simulink model "w3_warplab_trigger_proc"  (Simulink 7.7)
settings: Solver=ode45  StartTime=0.0  StopTime=100  RelTol=1e-3
InitFcn:
  | warplab_trigger_proc_init
StartFcn:
  | warplab_trigger_proc_init
undefined symbols (not defined in the file or in its folder): gcbh, xlBlockLoadCallback, xlGetNormalizedPeriod
libraries: xbsIndex_r4 x817, xbsEDKLib_r4 x1
(part 1 of 6)
settings Model: Creator=murphpo  LastModifiedBy=chunter
settings DebuggingCC: FcnCallInpInsideContextMsg=Enable All

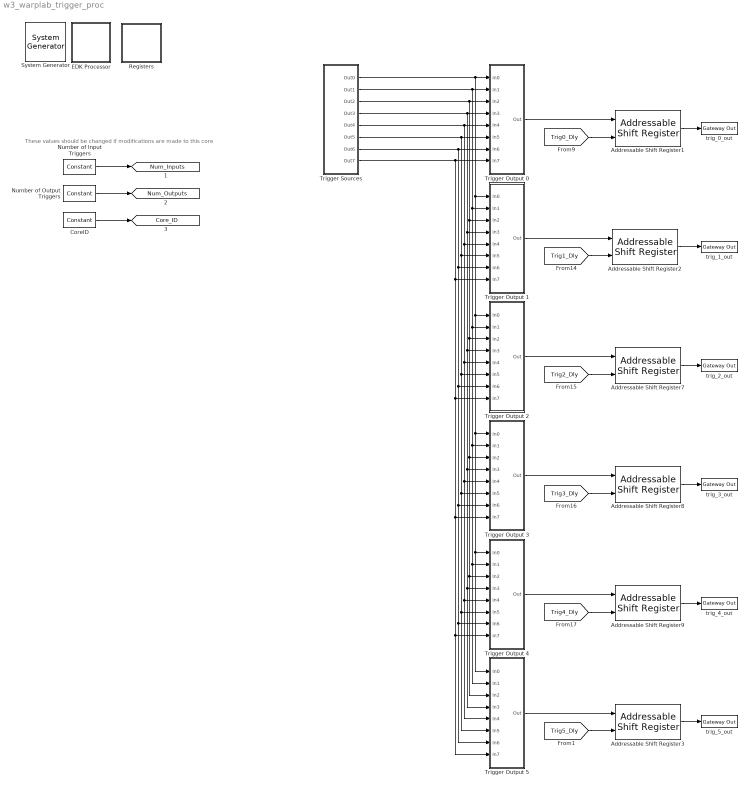
== system w3_warplab_trigger_proc ==
  note: These values should be changed if modifications are made to this core
  " System Generator" : xbsIndex_r4/ System Generator  Tag=genX  SystemSampleTime=-1  xilinxfamily=virtex6  part=xc6vlx240t  speed=-2  package=ff1156  synthesis_tool=XST  clock_wrapper=Clock Enables  directory=./netlist  proj_type=Project Navigator  Synth_file=XST Defaults  Impl_file=ISE Defaults  testbench=off  simulink_period=1  sysclk_period=10  dcm_input_clock_period=10  incr_netlist=off  trim_vbits=Everywhere in SubSystem  dbl_ovrd=According to Block Masks  core_generation=According to Block Masks  run_coregen=off  deprecated_control=off  eval_field=0  block_type=sysgen
  Addressable Shift Register{1..3,7..9} (6 alike) : xbsIndex_r4/Addressable Shift Register  infer_latency=off  depth=32  initVector=[0]  en=off  dbl_ovrd=off  use_behavioral_HDL=off  Optimization=Resource  block_type=addrsr
      settings: infoedit="Delay of configurable length.  Any element in the delay line can be addressed and driven onto the output port.<br><br>Hardware notes: This block is implemented using SRL16s. If Virtex-4 or Spartan-3 device is used, multiple SRLC16s are cascaded together."
  CoreID : xbsIndex_r4/Constant  const=0  gui_display_data_type=Fixed-point  arith_type=Unsigned  n_bits=8  bin_pt=0  preci_type=Single  exp_width=8  frac_width=24  explicit_period=on  period=1  equ=P=C  opselect=C  inp2=PCIN>>17  opr=+  inp1=P  carry=CIN  dbl_ovrd=off  block_type=constant
  EDK Processor : Subsystem  LoadFcn=xlBlockLoadCallback(gcbh);  mask(Xilinx EDK Processor Block){mode=EDK pcore generation, xmp=, MemVisToProc=<qt bgcolor="#FFFFFF"><div><img src="C:/Xilinx/14.4/ISE_DS/ISE/sysgen/data/images/registerplus.gif"> &lt;&lt;RSSI_PKT_DET_CONFIG&gt;&gt;<br></div><div><img src="C:/Xilinx/14.4/ISE_DS/ISE/sysgen/data/images/registerplus.gif"> &lt;&lt;TRIG_CONF_OUT5&gt;&gt;<br></div><div><img src="C:/Xilinx/14.4/ISE_DS/ISE/sysgen/data/images/registerplus.gif"> &lt;&lt;TRIG_CONF_OUT4&gt;&gt;<br></div><div><img src="C:/Xilinx/14.4/ISE_DS/ISE/sysgen/data/images/registerplus.gif"> &lt;&lt;TRIG_CONF_OUT3&gt;&gt;<br></div><div><img src="C:/Xilinx/14.4/ISE_DS/ISE/sysgen/data/images/registerplus.gif"> &lt;&lt;TRIG_CONF_OUT2&gt;&gt;<br></div><div><img src="C:/Xilinx/14.4/ISE_DS/ISE/sysgen/data/images/registerplus.gif"> &lt;&lt;TRIG_CONF_OUT1&gt;&gt;<br></div><div><img src="C:/Xilinx/14.4/ISE_DS/ISE/sysgen/data/images/registerplus.gif"> &lt;&lt;TRIG_CONF_OUT0&gt;&gt;<br></div><div><img src="C:/Xilinx/14.4/ISE_DS/ISE/sysgen/data/images/registerplus.gif"> &lt;&lt;RSSI_PKT_DET_DURATIONS&gt;&gt;<br></div><div><img src="C:/Xilinx/14.4/ISE_DS/ISE/sysgen/data/images/registerplus.gif"> &lt;&lt;RSSI_PKT_DET_THRESHOLDS&gt;&gt;<br></div><div><img src="C:/Xilinx/14.4/ISE_DS/ISE/sysgen/data/images/registerplus.gif"> &lt;&lt;TRIG_CONF_INBANK0&gt;&gt;<br></div><div><img src="C:/Xilinx/14.4/ISE_DS/ISE/sysgen/data/images/registerplus.gif"> &lt;&lt;TRIG_CONF_INBANK1&gt;&gt;<br></div><div><img src="C:/Xilinx/14.4/ISE_DS/ISE/sysgen/data/images/registerplus.gif"> &lt;&lt;CORE_INFO&gt;&gt;<br></div><div><img src="C:/Xilinx/14.4/ISE_DS/ISE/sysgen/data/images/registerplus.gif"> &lt;&lt;TRIG_OUT&gt;&gt;<br></div><div><img src="C:/Xilinx/14.4/ISE_DS/ISE/sysgen/data/images/memoryplus.gif"> &lt;&lt;PktOps0&gt;&gt;<br></div><div><img src="C:/Xilinx/14.4/ISE_DS/ISE/sysgen/data/images/memoryplus.gif"> &lt;&lt;PktTemplate0&gt;&gt;<br></div></qt>, AvailableMemories=<empty>, portInterfaceTable={'exposed'=>[],'portdir'=>[],'portname'=>[],'shortname'=>[]}, bus_type_sgadvanced=, bus_type=AXI, baseaddr=0x80000000, baseaddr_lock_sgadvanced=, baseaddr_lock=off, dual_clock_sgadvanced=, dual_clock=on, reg_readback_sgadvanced=, reg_readback=on, ucf_file=, inheritDeviceType_sgadvanced=, inheritDeviceType=off, elf_file=, codebug_sgadvanced=, codebug=on, clock_name=plb, internalPortList={}, resetPolarity=0, memxtable={'mladdr'=>[0.00000000000000000,1.00000000000000000,2.00000000000000000,3.00000000000000000,4.00000000000000000,5.00000000000000000,6.00000000000000000,7.00000000000000000,8.00000000000000000,9.00000000000000000,10.00000000000000000,0.00000000000000000,1.00000000000000000,-1.00000000000000000,-1.00000000000000000],'mlist'=>['w3_warplab_trigger_proc/Registers/From Register9','w3_warplab_trigger_proc/Registers/From Register7','w3_warplab_trigger_proc/Registers/From Register6','w3_warplab_trigger_proc/Registers/From Register5','w3_warplab_trigger_proc/Registers/From Register4','w3_warplab_trigger_proc/Registers/From Register3','w3_warplab_trigger_proc/Registers/From Register2','w3_warplab_trigger_proc/Registers/From Register11','w3_warplab_trigger_proc/Registers/From Register10','w3_warplab_trigger_proc/Registers/From Register1','w3_warplab_trigger_proc/Registers/From Register','w3_warplab_trigger_proc/Registers/To Register1','w3_warplab_trigger_proc/Registers/To Register','w3_warplab_trigger_proc/Trigger Sources/Ethernet/Pkt Comp/Word Comp 0/Shared Memory2','w3_warplab_trigger_proc/Trigger Sources/Ethernet/Pkt Comp/Word Comp 0/Shared Memory1'],'mlname'=>['\\'RSSI_PKT_DET_CONFIG\\'','\\'TRIG_CONF_OUT5\\'','\\'TRIG_CONF_OUT4\\'','\\'TRIG_CONF_OUT3\\'','\\'TRIG_CONF_OUT2\\'','\\'TRIG_CONF_OUT1\\'','\\'TRIG_CONF_OUT0\\'','\\'RSSI_PKT_DET_DURATIONS\\'','\\'RSSI_PKT_DET_THRESHOLDS\\'','\\'TRIG_CONF_INBANK0\\'','\\'TRIG_CONF_INBANK1\\'','\\'CORE_INFO\\'','\\'TRIG_OUT\\'','\\'PktOps0\\'','\\'PktTemplate0\\''],'mlstate'=>[0.00000000000000000,0.00000000000000000,0.00000000000000000,0.00000000000000000,0.00000000000000000,0.00000000000000000,0.00000000000000000,0.00000000000000000,0.00000000000000000,0.00000000000000000,0.00000000000000000,0.00000000000000000,0.00000000000000000,0.00000000000000000,0.00000000000000000]}, procinfo={}, memmapdirty=off, blockname=, xpsintstyle=default, has_advanced_control=0, sggui_pos=-1,-1,-1,-1, block_type=edkprocessor, block_version=2.7, sg_icon_stat=62,64,-1,-1,white,blue,0,07734,right,,[ ],[ ], sg_mask_display=|, sg_list_contents={'table'=>{'AvailableMemories'=>'popup(<empty>)'}}, sg_blockgui_xml=}
      mask sg_mask_display=|
      | fprintf('','COMMENT: begin icon graphics');
      | patch([0 62 62 0 0 ],[0 0 64 64 0 ],[0.77 0.82 0.91 ]);
      | plot([0 62 62 0 0 ],[0 0 64 64 0 ]);
      | patch([13.2 24.76 32.76 40.76 48.76 32.76 21.2 13.2 ],[40.88 40.88 48.88 40.88 48.88 48.88 48.88 40.88 ],[1 1 1 ]);
      | patch([21.2 32.76 24.76 13.2 21.2 ],[32.88 32.88 40.88 40.88 32.88 ],[0.931 0.946 0.973 ]);
      | patch([13.2 24.76 32.76 21.2 13.2 ],[24.88 24.88 32.88 32.88 24.88 ],[1 1 1 ]);
      | patch([21.2 48.76 40.76 32.76 24.76 13.2 21.2 ],[16.88 16.88 24.88 16.88 24.88 24.88 16.88 ],[0.931 0.946 0.973 ]);
      | fprintf('','COMMENT: end icon graphics');
      | fprintf('','COMMENT: begin icon text');
      | fprintf('','COMMENT: end icon text');
      mask prompts: mode "Configure Processor for"; xmp "XPS Project"; MemVisToProc ""; AvailableMemories "Available Memories"; portInterfaceTable ""; bus_type_sgadvanced ""; bus_type "Bus Type"; baseaddr "Base Address"; baseaddr_lock_sgadvanced ""; baseaddr_lock "Lock"; dual_clock_sgadvanced ""; dual_clock "Dual Clocks"; reg_readback_sgadvanced ""; reg_readback "Register Read-Back"; ucf_file "Constraint File"; inheritDeviceType_sgadvanced ""; inheritDeviceType "Inherit Device Type"; elf_file "Initial Program"; codebug_sgadvanced ""; codebug "Enable Co-Debug with Xilinx SDK (Beta)"; clock_name ""; internalPortList ""; resetPolarity ""; memxtable ""; procinfo ""; memmapdirty ""; blockname ""; xpsintstyle ""; has_advanced_control ""; sggui_pos ""; block_type ""; block_version ""; sg_icon_stat ""; sg_mask_display ""; sg_list_contents ""; sg_blockgui_xml ""
      mask help: Xilinx EDK Processor
      mask init:
      | try
      |   tmp_gcb = gcb;
      |   tmp_gcbh = gcbh;
      |   if (strcmp('SysGenIndex',get_param(bdroot(tmp_gcbh),'tag')) && ~isempty(regexp(bdroot(tmp_gcb), '^xbs', 'once')))
      |     return;
      |   end;
      |   xlMungeMaskParams;
      | 
      |   block_type='edkprocessor';
      | 
      |   serialized_declarations = '{''block_type''=>''String''}';
      |   xledkprocessor_init();
      |   ptable_ = xlblockprep(get_param(tmp_gcb, 'MaskWSVariables'));
      |   try
      |     xlBlockMoveCallback(tmp_gcbh);
      |   catch 
      |      clear global xl_updateicon_recursion_guard;
      |   end;
      | catch
      |   global dbgsysgen;
      |   if(~isempty(dbgsysgen) && dbgsysgen)
      |     e = regexprep(lasterr, '\n', '\nError: ');
      |     disp(['Error: While running MaskInit code on block ' tmp_gcb ': ' e]);
      |     error(e);
      |   end
      | end
      settings: CopyFcn=xlProcBlockCopyCallback(gcbh);xlBlockMoveCallback(gcbh);  DeleteFcn=xlDestroyGui(gcbh);  ModelCloseFcn=xlDestroyGui(gcbh);  PreSaveFcn=xlBlockPreSaveCallback(gcbh);  PostSaveFcn=xlBlockPostSaveCallback(gcbh);  DestroyFcn=xlDestroyGui(gcbh);  OpenFcn=bh=gcbh;xlProcBlockCallbacks('populatesharedmemorylistbox',bh);xlOpenGui(bh, 'edkprocessor_gui.xml', @xlProcBlockEnablement, @xlProcBlockAction);  CloseFcn=xlDestroyGui(gcbh);  MoveFcn=xlBlockMoveCallback(gcbh);
      mask Help: eval('');xlDoc('-book','sysgen','-topic','EDK_Processor');
      mask StyleString: popup(EDK pcore generation|HDL netlisting),edit,edit,edit,edit,edit,popup(AXI|PLB),edit,edit,checkbox,edit,checkbox,edit,checkbox,edit,edit,checkbox,edit,edit,checkbox,edit,edit,edit,edit,edit,edit,edit,edit,edit,edit,edit,edit,edit,edit,edit,edit
      mask Display:
      | fprintf('','COMMENT: begin icon graphics');
      | patch([0 62 62 0 0 ],[0 0 64 64 0 ],[0.77 0.82 0.91 ]);
      | plot([0 62 62 0 0 ],[0 0 64 64 0 ]);
      | patch([13.2 24.76 32.76 40.76 48.76 32.76 21.2 13.2 ],[40.88 40.88 48.88 40.88 48.88 48.88 48.88 40.88 ],[1 1 1 ]);
      | patch([21.2 32.76 24.76 13.2 21.2 ],[32.88 32.88 40.88 40.88 32.88 ],[0.931 0.946 0.973 ]);
      | patch([13.2 24.76 32.76 21.2 13.2 ],[24.88 24.88 32.88 32.88 24.88 ],[1 1 1 ]);
      | patch([21.2 48.76 40.76 32.76 24.76 13.2 21.2 ],[16.88 16.88 24.88 16.88 24.88 24.88 16.88 ],[0.931 0.946 0.973 ]);
      | fprintf('','COMMENT: end icon graphics');
      | fprintf('','COMMENT: begin icon text');
      | disp('');
      | 
      | fprintf('','COMMENT: end icon text');
  Number of Input Triggers : xbsIndex_r4/Constant  const=8  gui_display_data_type=Fixed-point  arith_type=Unsigned  n_bits=8  bin_pt=0  preci_type=Single  exp_width=8  frac_width=24  explicit_period=on  period=1  equ=P=C  opselect=C  inp2=PCIN>>17  opr=+  inp1=P  carry=CIN  dbl_ovrd=off  block_type=constant
  Number of Output Triggers : xbsIndex_r4/Constant  const=6  gui_display_data_type=Fixed-point  arith_type=Unsigned  n_bits=8  bin_pt=0  preci_type=Single  exp_width=8  frac_width=24  explicit_period=on  period=1  equ=P=C  opselect=C  inp2=PCIN>>17  opr=+  inp1=P  carry=CIN  dbl_ovrd=off  block_type=constant
  Registers : Subsystem
  Trigger Output 0 : Subsystem
  Trigger Output 1 : Subsystem
  Trigger Output 2 : Subsystem
  Trigger Output 3 : Subsystem
  Trigger Output 4 : Subsystem
  Trigger Output 5 : Subsystem
  Trigger Sources : Subsystem
  trig_0_out : xbsIndex_r4/Gateway Out  inherit_from_input=off  hdl_port=on  timing_constraint=None  locs_specified=off  LOCs={}  UseAsDAC=off  DACChannel='1'  block_type=gatewayout
  trig_1_out : xbsIndex_r4/Gateway Out  inherit_from_input=off  hdl_port=on  timing_constraint=None  locs_specified=off  LOCs={}  UseAsDAC=off  DACChannel='1'  block_type=gatewayout
  trig_2_out : xbsIndex_r4/Gateway Out  inherit_from_input=off  hdl_port=on  timing_constraint=None  locs_specified=off  LOCs={}  UseAsDAC=off  DACChannel='1'  block_type=gatewayout
  trig_3_out : xbsIndex_r4/Gateway Out  inherit_from_input=off  hdl_port=on  timing_constraint=None  locs_specified=off  LOCs={}  UseAsDAC=off  DACChannel='1'  block_type=gatewayout
  trig_4_out : xbsIndex_r4/Gateway Out  inherit_from_input=off  hdl_port=on  timing_constraint=None  locs_specified=off  LOCs={}  UseAsDAC=off  DACChannel='1'  block_type=gatewayout
  trig_5_out : xbsIndex_r4/Gateway Out  inherit_from_input=off  hdl_port=on  timing_constraint=None  locs_specified=off  LOCs={}  UseAsDAC=off  DACChannel='1'  block_type=gatewayout
  tag scope: Core_ID=global, Num_Inputs=global, Num_Outputs=global
  wires:
  Trigger Sources/1(Out0) -> Trigger Output 0/1(In0), Trigger Output 3/1(In0), Trigger Output 4/1(In0), Trigger Output 5/1(In0), Trigger Output 2/1(In0), Trigger Output 1/1(In0)
  Trigger Sources/2(Out1) -> Trigger Output 0/2(In1), Trigger Output 3/2(In1), Trigger Output 4/2(In1), Trigger Output 5/2(In1), Trigger Output 2/2(In1), Trigger Output 1/2(In1)
  Trigger Sources/3(Out2) -> Trigger Output 0/3(In2), Trigger Output 3/3(In2), Trigger Output 4/3(In2), Trigger Output 5/3(In2), Trigger Output 2/3(In2), Trigger Output 1/3(In2)
  Trigger Sources/4(Out3) -> Trigger Output 0/4(In3), Trigger Output 3/4(In3), Trigger Output 4/4(In3), Trigger Output 5/4(In3), Trigger Output 2/4(In3), Trigger Output 1/4(In3)
  Trigger Sources/5(Out4) -> Trigger Output 0/5(In4), Trigger Output 3/5(In4), Trigger Output 4/5(In4), Trigger Output 5/5(In4), Trigger Output 2/5(In4), Trigger Output 1/5(In4)
  Trigger Sources/6(Out5) -> Trigger Output 0/6(In5), Trigger Output 3/6(In5), Trigger Output 4/6(In5), Trigger Output 5/6(In5), Trigger Output 2/6(In5), Trigger Output 1/6(In5)
  Trigger Sources/7(Out6) -> Trigger Output 0/7(In6), Trigger Output 3/7(In6), Trigger Output 4/7(In6), Trigger Output 5/7(In6), Trigger Output 2/7(In6), Trigger Output 1/7(In6)
  Trigger Sources/8(Out7) -> Trigger Output 0/8(In7), Trigger Output 3/8(In7), Trigger Output 4/8(In7), Trigger Output 5/8(In7), Trigger Output 2/8(In7), Trigger Output 1/8(In7)
  Trigger Output 0/1(Out) -> Addressable Shift Register1/1
  Addressable Shift Register1/1 -> trig_0_out/1
  Trigger Output 1/1(Out) -> Addressable Shift Register2/1
  Addressable Shift Register2/1 -> trig_1_out/1
  Trigger Output 2/1(Out) -> Addressable Shift Register7/1
  Addressable Shift Register7/1 -> trig_2_out/1
  Trigger Output 3/1(Out) -> Addressable Shift Register8/1
  Addressable Shift Register8/1 -> trig_3_out/1
  Trigger Output 4/1(Out) -> Addressable Shift Register9/1
  Addressable Shift Register9/1 -> trig_4_out/1
  [Trig0_Dly] -> Addressable Shift Register1/2
  [Trig1_Dly] -> Addressable Shift Register2/2
  [Trig2_Dly] -> Addressable Shift Register7/2
  [Trig3_Dly] -> Addressable Shift Register8/2
  [Trig4_Dly] -> Addressable Shift Register9/2
  Number of Input Triggers/1 -> [Num_Inputs]
  Number of Output Triggers/1 -> [Num_Outputs]
  CoreID/1 -> [Core_ID]
  Trigger Output 5/1(Out) -> Addressable Shift Register3/1
  Addressable Shift Register3/1 -> trig_5_out/1
  [Trig5_Dly] -> Addressable Shift Register3/2
